simulink model "mrastate"  (R2013a)
settings: Solver=ode5  StartTime=0.0  StopTime=20  FixedStep=1e-3  RelTol=1e-6
undefined symbols (not defined in the file): b, k, m
settings Model: Creator=windows 10  LastModifiedBy=windows 10

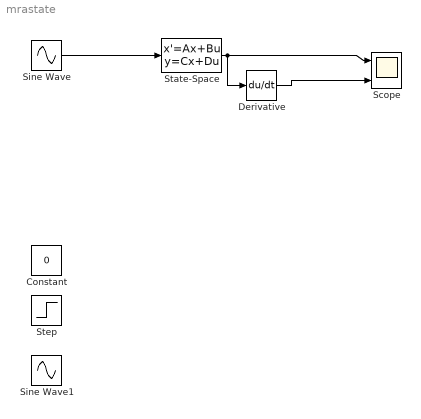
== system mrastate ==
  Constant : Constant  Value=0
  Derivative : Derivative
  Scope : Scope  NumInputPorts=2
      settings: YMin=-5~-5  YMax=5~5
  Sine Wave : Sin  Amplitude=2  Phase=pi/2  SampleTime=0
  Sine Wave1 : Sin  Amplitude=2  Frequency=8*pi  Phase=pi/2  SampleTime=0
  State-Space : StateSpace  A=[0 1; -k/m -b/m]  B=[0;1/m]  C=[1 0]  D=0  X0=[1 0]
  Step : Step  Time=0  After=5  SampleTime=0
  wires:
  State-Space/1 -> Derivative/1, Scope/1
  Derivative/1 -> Scope/2
  Sine Wave/1 -> State-Space/1
